simulink model "districtResourceModel"  (R2026a)
settings: Solver=FixedStepDiscrete  StopTime=inf  FixedStep=60
model workspace (MAT data in the model file):
  AnnualPatients = 100000
  BandwidthMbps = [0.5 1 2 5]
  ImageSizeMB = 4
  NumOphthalmologists = 2
  NumPhcs = 10
  ReviewSecondsB = 30
  ReviewSecondsC = 240
  RngSeed = 42
  SimDays = 20
  TierFractions = [0.384 0.438 0.178]
  WorkingDaysPerYear = 250
  WorkingHoursPerDay = 8
settings Model: Creator=91740  LastModifiedBy=91740

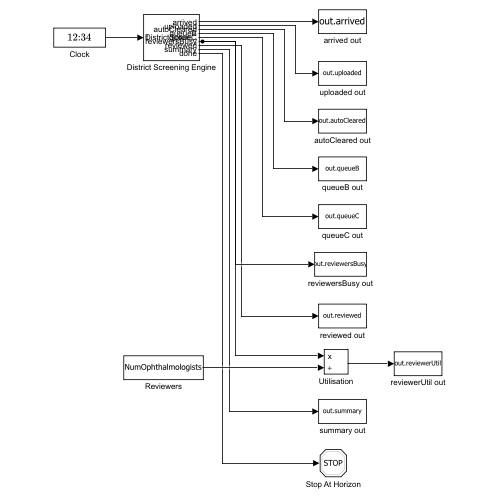
[thumbnail: Simulink's stored preview of the top-level diagram]
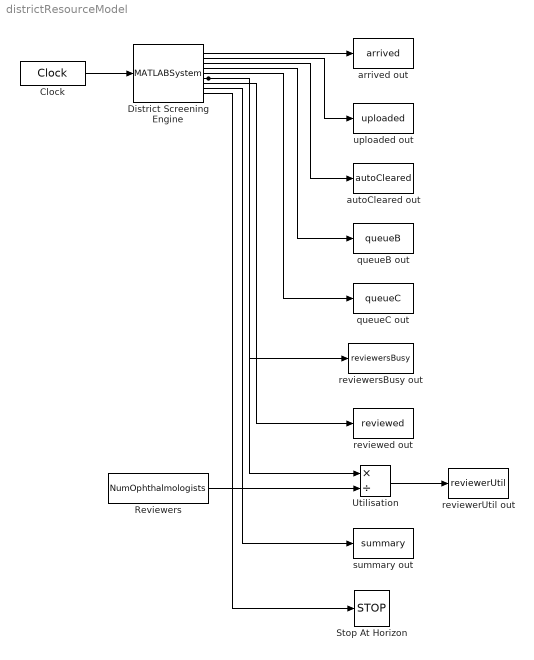
== system districtResourceModel ==
  Clock : DigitalClock  SampleTime=60
  District Screening Engine : MATLABSystem  System=DistrictScreeningEngine  AnnualPatients=AnnualPatients  NumPhcs=NumPhcs  WorkingDaysPerYear=WorkingDaysPerYear  WorkingHoursPerDay=WorkingHoursPerDay  ImageSizeMB=ImageSizeMB  BandwidthMbps=BandwidthMbps  NumOphthalmologists=NumOphthalmologists  TierFractions=TierFractions  ReviewSecondsB=ReviewSecondsB  ReviewSecondsC=ReviewSecondsC  SimDays=SimDays  RngSeed=RngSeed  MaxCases=500000  MaxReviewers=20  MaxPhcs=200  SimulateUsing=Code generation
      mask Type: DistrictScreeningEngine
  Reviewers : Constant  Value=NumOphthalmologists  SampleTime=60
  Stop At Horizon : Stop
  Utilisation : Product  Inputs=*/
  arrived out : ToWorkspace  VariableName=arrived  SaveFormat=Timeseries  SampleTime=-1
  autoCleared out : ToWorkspace  VariableName=autoCleared  SaveFormat=Timeseries  SampleTime=-1
  queueB out : ToWorkspace  VariableName=queueB  SaveFormat=Timeseries  SampleTime=-1
  queueC out : ToWorkspace  VariableName=queueC  SaveFormat=Timeseries  SampleTime=-1
  reviewed out : ToWorkspace  VariableName=reviewed  SaveFormat=Timeseries  SampleTime=-1
  reviewerUtil out : ToWorkspace  VariableName=reviewerUtil  SaveFormat=Timeseries  SampleTime=-1
  reviewersBusy out : ToWorkspace  VariableName=reviewersBusy  SaveFormat=Timeseries  SampleTime=-1
  summary out : ToWorkspace  VariableName=summary  SaveFormat=Timeseries  SampleTime=-1
  uploaded out : ToWorkspace  VariableName=uploaded  SaveFormat=Timeseries  SampleTime=-1
  wires:
  Clock/1 -> District Screening Engine/1
  District Screening Engine/1 -> arrived out/1
  District Screening Engine/5 -> queueC out/1
  District Screening Engine/4 -> queueB out/1
  District Screening Engine/3 -> autoCleared out/1
  District Screening Engine/2 -> uploaded out/1
  District Screening Engine/7 -> reviewed out/1
  District Screening Engine/6 -> Utilisation/1, reviewersBusy out/1
  District Screening Engine/8 -> summary out/1
  District Screening Engine/9 -> Stop At Horizon/1
  Reviewers/1 -> Utilisation/2
  Utilisation/1 -> reviewerUtil out/1
